simulink model "ksrbl_4k4t_hdtrig"  (Simulink 6.2)
settings: Solver=ode45  StartTime=0.0  StopTime=20000  RelTol=1e-3
libraries: xbsIndex_r3 x1214, casper_library x120, xps_library x20
(part 25 of 26)

== system ksrbl_4k4t_hdtrig/fft_wideband_real/fft_biplex_real_4x0/biplex_core/fft_stage_9/butterfly_direct ==
  a : Inport  Port=1  LatchInput=off
  b : Inport  Port=2  LatchInput=off
  sync : Inport  Port=3  LatchInput=off
  shift : Inport  Port=4  LatchInput=off
  AddSub : xbsIndex_r3/AddSub  mode=Addition  precision=Full  arith_type=Unsigned  n_bits=8  bin_pt=2  quantization=Truncate  overflow=Wrap  latency=add_latency  explicit_period=off  period=1  use_carryin=off  use_carryout=off  en=off  dbl_ovrd=off  show_param=on  use_core=on  pipeline=on  use_rpm=on  gen_core=on
      settings: xl_area=[0, 0, 0, 0, 0, 0, 0]
  AddSub1 : xbsIndex_r3/AddSub  mode=Addition  precision=Full  arith_type=Unsigned  n_bits=8  bin_pt=2  quantization=Truncate  overflow=Wrap  latency=add_latency  explicit_period=off  period=1  use_carryin=off  use_carryout=off  en=off  dbl_ovrd=off  show_param=on  use_core=on  pipeline=on  use_rpm=on  gen_core=on
      settings: xl_area=[0, 0, 0, 0, 0, 0, 0]
  AddSub2 : xbsIndex_r3/AddSub  mode=Subtraction  precision=Full  arith_type=Unsigned  n_bits=8  bin_pt=2  quantization=Truncate  overflow=Wrap  latency=add_latency  explicit_period=off  period=1  use_carryin=off  use_carryout=off  en=off  dbl_ovrd=off  show_param=on  use_core=on  pipeline=on  use_rpm=on  gen_core=on
      settings: xl_area=[0, 0, 0, 0, 0, 0, 0]
  AddSub3 : xbsIndex_r3/AddSub  mode=Subtraction  precision=Full  arith_type=Unsigned  n_bits=8  bin_pt=2  quantization=Truncate  overflow=Wrap  latency=add_latency  explicit_period=off  period=1  use_carryin=off  use_carryout=off  en=off  dbl_ovrd=off  show_param=on  use_core=on  pipeline=on  use_rpm=on  gen_core=on
      settings: xl_area=[0, 0, 0, 0, 0, 0, 0]
  Convert{,1..3} (4 alike) : xbsIndex_r3/Convert  arith_type="Signed  (2's comp)"  n_bits=BitWidth  bin_pt=BitWidth-1  quantization=Truncate  overflow=Wrap  latency=add_latency  explicit_period=off  period=1  dbl_ovrd=off  show_param=off  inserted_by_tool=off  pipeline=off
      settings: xl_area=[0, 0, 0, 0, 0, 0, 0]
  Delay : xbsIndex_r3/Delay  latency=2 * add_latency + 1  reg_retiming=off  explicit_period=off  period=1  en=off  accept_only_valid=off  init_zero=on  dbl_ovrd=off  show_param=off
      settings: xl_area=[0, 0, 0, 0, 0, 0, 0]
  Delay3 : xbsIndex_r3/Delay  latency=1  reg_retiming=off  explicit_period=off  period=1  en=off  accept_only_valid=off  init_zero=on  dbl_ovrd=off  show_param=off
      settings: xl_area=[0, 0, 0, 0, 0, 0, 0]
  Inverter : xbsIndex_r3/Inverter  latency=0  explicit_period=off  period=1  en=off  dbl_ovrd=off  show_param=off
      settings: xl_area=[0, 0, 0, 0, 0, 0, 0]
  Logical : xbsIndex_r3/Logical  logical_function=OR  inputs=4  precision=Full  arith_type=Unsigned  n_bits=8  bin_pt=2  align_bp=on  latency=1  explicit_period=off  period=1  en=off  dbl_ovrd=off  show_param=off
      settings: xl_area=[0, 0, 0, 0, 0, 0, 0]
  Logical{1,4,7,10} (4 alike) : xbsIndex_r3/Logical  logical_function=OR  inputs=2  precision=Full  arith_type=Unsigned  n_bits=8  bin_pt=2  align_bp=off  latency=1  explicit_period=off  period=1  en=off  dbl_ovrd=off  show_param=off
      settings: xl_area=[0, 0, 0, 0, 0, 0, 0]
  Logical{2,5,8,11} (4 alike) : xbsIndex_r3/Logical  logical_function=NOR  inputs=4  precision=Full  arith_type=Unsigned  n_bits=8  bin_pt=2  align_bp=off  latency=1  explicit_period=off  period=1  en=off  dbl_ovrd=off  show_param=off
      settings: xl_area=[0, 0, 0, 0, 0, 0, 0]
  Logical{3,6,9,12} (4 alike) : xbsIndex_r3/Logical  logical_function=AND  inputs=4  precision=Full  arith_type=Unsigned  n_bits=8  bin_pt=2  align_bp=off  latency=1  explicit_period=off  period=1  en=off  dbl_ovrd=off  show_param=off
      settings: xl_area=[0, 0, 0, 0, 0, 0, 0]
  Logical13 : xbsIndex_r3/Logical  logical_function=AND  inputs=2  precision=Full  arith_type=Unsigned  n_bits=8  bin_pt=2  align_bp=off  latency=1  explicit_period=off  period=1  en=off  dbl_ovrd=off  show_param=off
      settings: xl_area=[0, 0, 0, 0, 0, 0, 0]
  Mux{,1..3} (4 alike) : xbsIndex_r3/Mux  inputs=2  precision=Full  arith_type="Signed  (2's comp)"  n_bits=8  bin_pt=2  quantization=Truncate  overflow=Wrap  latency=1  explicit_period=off  period=1  en=off  dbl_ovrd=off  show_param=off  mux_type=off  use_rpm=off  gen_core=off
      settings: xl_area=[0, 0, 0, 0, 0, 0, 0]
  Scale{,1..3} (4 alike) : xbsIndex_r3/Scale  scale_factor=-1  explicit_period=off  period=1  dbl_ovrd=off
  Slice{1,5,9,13} (4 alike) : xbsIndex_r3/Slice  mode=Upper Bit Location + Width  nbits=1  bit1=0  base1=MSB of Input  bit0=0  base0=LSB of Input  boolean_output=on  explicit_period=off  period=1  dbl_ovrd=off
  Slice{2,6,10,14} (4 alike) : xbsIndex_r3/Slice  mode=Upper Bit Location + Width  nbits=1  bit1=-1  base1=MSB of Input  bit0=0  base0=LSB of Input  boolean_output=on  explicit_period=off  period=1  dbl_ovrd=off
  Slice{3,7,11,15} (4 alike) : xbsIndex_r3/Slice  mode=Upper Bit Location + Width  nbits=1  bit1=-2  base1=MSB of Input  bit0=0  base0=LSB of Input  boolean_output=on  explicit_period=off  period=1  dbl_ovrd=off
  Slice{4,8,12,16} (4 alike) : xbsIndex_r3/Slice  mode=Upper Bit Location + Width  nbits=1  bit1=-3  base1=MSB of Input  bit0=0  base0=LSB of Input  boolean_output=on  explicit_period=off  period=1  dbl_ovrd=off
  ri_to_c : casper_library/Misc/ri_to_c
  ri_to_c1 : casper_library/Misc/ri_to_c
  twiddle : Subsystem  BlockChoice=twiddle_general_3mult
      link override twiddle_general_3mult: Coeffs="[1+0i           6.1232e-017-1i               0.70711-0.70711i        -0.70711-0.70711i         0.92388-0.38268i        -0.38268-0.92388i         0.38268-0.92388i        -0.92388-0.38268i         0.98079-0.19509i        -0.19509-0.98079i         0.55557-0.83147i        -0.83147-0.55557i         0.83147-0.55557i        -0.55557-0.83147i         0.19509-0.98079i        -0.98079-0.19509i         0.99518-0.098017i      -0.098017-0.99518i         0.63439-0.77301i        -0.77301-0.63439i         0.88192-0.4714i          -0.4714-0.88192i         0.29028-0.95694i        -0.95694-0.29028i         0.95694-0.29028i        -0.29028-0.95694i          0.4714-0.88192i        -0.88192-0.4714i          0.77301-0.63439i        -0.63439-0.77301i        0.098017-0.99518i        -0.99518-0.098017i         0.9988-0.049068i      -0.049068-0.9988i          0.67156-0.74095i        -0.74095-0.67156i         0.90399-0.42756i        -0.42756-0.90399i         0.33689-0.94154i        -0.94154-0.33689i         0.97003-0.24298i        -0.24298-0.97003i          0.5141-0.85773i        -0.85773-0.5141i          0.80321-0.5957i          -0.5957-0.80321i         0.14673-0.98918i        -0.98918-0.14673i         0.98918-0.14673i        -0.14673-0.98918i          0.5957-0.80321i        -0.80321-0.5957i          0.85773-0.5141i          -0.5141-0.85773i         0.24298-0.97003i        -0.97003-0.24298i         0.94154-0.33689i        -0.33689-0.94154i         0.42756-0.90399i        -0.90399-0.42756i         0.74095-0.67156i        -0.67156-0.74095i        0.049068-0.9988i          -0.9988-0.049068i         0.9997-0.024541i      -0.024541-0.9997i          0.68954-0.72425i        -0.72425-0.68954i         0.91421-0.40524i        -0.40524-0.91421i          0.3599-0.93299i        -0.93299-0.3599i           0.9757-0.2191i          -0.2191-0.9757i            0.535-0.84485i        -0.84485-0.535i           0.81758-0.57581i        -0.57581-0.81758i         0.17096-0.98528i        -0.98528-0.17096i         0.99248-0.12241i        -0.12241-0.99248i         0.61523-0.78835i        -0.78835-0.61523i         0.87009-0.4929i          -0.4929-0.87009i         0.26671-0.96378i        -0.96378-0.26671i         0.94953-0.31368i        -0.31368-0.94953i         0.44961-0.89322i        -0.89322-0.44961i         0.75721-0.65317i        -0.65317-0.75721i        0.073565-0.99729i        -0.99729-0.073565i        0.99729-0.073565i      -0.073565-0.99729i         0.65317-0.75721i        -0.75721-0.65317i         0.89322-0.44961i        -0.44961-0.89322i         0.31368-0.94953i        -0.94953-0.31368i         0.96378-0.26671i        -0.26671-0.96378i          0.4929-0.87009i        -0.87009-0.4929i          0.78835-0.61523i        -0.61523-0.78835i         0.12241-0.99248i        -0.99248-0.12241i         0.98528-0.17096i        -0.17096-0.98528i         0.57581-0.81758i        -0.81758-0.57581i         0.84485-0.535i            -0.535-0.84485i          0.2191-0.9757i          -0.9757-0.2191i          0.93299-0.3599i          -0.3599-0.93299i         0.40524-0.91421i        -0.91421-0.40524i         0.72425-0.68954i        -0.68954-0.72425i        0.024541-0.9997i          -0.9997-0.024541i        0.99992-0.012272i      -0.012272-0.99992i         0.69838-0.71573i        -0.71573-0.69838i         0.91911-0.39399i        -0.39399-0.91911i         0.37132-0.92851i        -0.92851-0.37132i         0.97832-0.20711i        -0.20711-0.97832i         0.54532-0.83822i        -0.83822-0.54532i         0.82459-0.56573i        -0.56573-0.82459i         0.18304-0.98311i        -0.98311-0.18304i         0.99391-0.11022i        -0.11022-0.99391i         0.62486-0.78074i        -0.78074-0.62486i         0.87607-0.48218i        -0.48218-0.87607i         0.27852-0.96043i        -0.96043-0.27852i         0.95331-0.30201i        -0.30201-0.95331i         0.46054-0.88764i        -0.88764-0.46054i         0.76517-0.64383i        -0.64383-0.76517i        0.085797-0.99631i        -0.99631-0.085797i ...(+2393 chars)   ]"  StepPeriod=1  BitWidth=18  add_latency=4  mult_latency=6  bram_latency=4
      link override twiddle_general_3mult/coeff_gen: BlockChoice=br_coeff_gen
      link override twiddle_general_3mult/coeff_gen/br_coeff_gen: Coeffs=[1 2 3 4 5 6 7]  StepPeriod=4  BitWidth=10  bram_latency=6
      link override twiddle_general_3mult/coeff_gen/br_coeff_gen/ROM: distributed_mem=off
      link override twiddle_general_3mult/coeff_gen/br_coeff_gen/ROM1: distributed_mem=off
      link override twiddle_general_3mult/coeff_gen/static_coeff_gen/Constant: equ=P=C
      link override twiddle_general_3mult/coeff_gen/static_coeff_gen/Constant1: equ=P=C
      settings: AttributesFormatString=%<BlockChoice>  TemplateBlock=casper_library/FFTs/Twiddle/twiddle  MemberBlocks=twiddle_coeff_0,twiddle_coeff_1,twiddle_general_3mult,twiddle_general_4mult,twiddle_stage_2
  a+bw : Outport
  a-bw : Outport  Port=2
  of : Outport  Port=3
  sync_out : Outport  Port=4
  wires:
  Inverter/1 -> Logical13/1
  Logical13/1 -> of/1
  Logical/1 -> Logical13/2
  Delay3/1 -> Inverter/1, Mux3/1, Mux2/1, Mux1/1, Mux/1
  Logical7/1 -> Logical/3
  AddSub3/1 -> Scale3/1, Mux3/2
  Logical10/1 -> Logical/4
  Logical11/1 -> Logical10/2
  Logical12/1 -> Logical10/1
  Slice16/1 -> Logical11/3, Logical11/4, Logical12/4
  Slice15/1 -> Logical12/3
  Slice14/1 -> Logical11/2, Logical12/2
  Slice13/1 -> Logical11/1, Logical12/1
  Convert3/1 -> ri_to_c1/2
  Scale3/1 -> Mux3/3
  Mux3/1 -> Slice16/1, Slice15/1, Slice14/1, Slice13/1, Convert3/1
  AddSub2/1 -> Scale2/1, Mux2/2
  Logical8/1 -> Logical7/2
  Logical9/1 -> Logical7/1
  Slice12/1 -> Logical8/4, Logical9/4
  Slice11/1 -> Logical8/3, Logical9/3
  Slice10/1 -> Logical8/2, Logical9/2
  Slice9/1 -> Logical8/1, Logical9/1
  Convert2/1 -> ri_to_c1/1
  Scale2/1 -> Mux2/3
  Mux2/1 -> Slice12/1, Slice11/1, Slice10/1, Slice9/1, Convert2/1
  Logical4/1 -> Logical/2
  Logical5/1 -> Logical4/2
  Logical6/1 -> Logical4/1
  Slice8/1 -> Logical5/3, Logical5/4, Logical6/4
  Slice7/1 -> Logical6/3
  Slice6/1 -> Logical5/2, Logical6/2
  Slice5/1 -> Logical5/1, Logical6/1
  Convert1/1 -> ri_to_c/2
  Scale1/1 -> Mux1/3
  Mux1/1 -> Slice8/1, Slice7/1, Slice6/1, Slice5/1, Convert1/1
  Logical1/1 -> Logical/1
  Logical2/1 -> Logical1/2
  Logical3/1 -> Logical1/1
  Slice4/1 -> Logical2/4, Logical3/4
  Slice3/1 -> Logical2/3, Logical3/3
  Slice2/1 -> Logical2/2, Logical3/2
  Slice1/1 -> Logical2/1, Logical3/1
  Convert/1 -> ri_to_c/1
  Scale/1 -> Mux/3
  Mux/1 -> Slice4/1, Slice3/1, Slice2/1, Slice1/1, Convert/1
  shift/1 -> Delay3/1
  AddSub1/1 -> Scale1/1, Mux1/2
  AddSub/1 -> Scale/1, Mux/2
  Delay/1 -> sync_out/1
  ri_to_c1/1 -> a-bw/1
  ri_to_c/1 -> a+bw/1
  a/1 -> twiddle/1(a)
  b/1 -> twiddle/2(b)
  sync/1 -> twiddle/3(sync)
  twiddle/1(a_re) -> AddSub/1, AddSub2/1
  twiddle/2(a_im) -> AddSub1/1, AddSub3/1
  twiddle/3(bw_re) -> AddSub/2, AddSub2/2
  twiddle/4(bw_im) -> AddSub1/2, AddSub3/2
  twiddle/5(sync_out) -> Delay/1

== system ksrbl_4k4t_hdtrig/fft_wideband_real/fft_biplex_real_4x0/biplex_core/fft_stage_9/delay_b ==
  In1 : Inport  Port=1  LatchInput=off
  delay_slr : casper_library/Delays/delay_slr  DelayLen=2^(FFTSize-FFTStage)
  Out1 : Outport
  wires:
  In1/1 -> delay_slr/1
  delay_slr/1 -> Out1/1

== system ksrbl_4k4t_hdtrig/fft_wideband_real/fft_biplex_real_4x0/biplex_core/fft_stage_9/delay_f ==
  In1 : Inport  Port=1  LatchInput=off
  delay_slr : casper_library/Delays/delay_slr  DelayLen=2^(FFTSize-FFTStage)
  Out1 : Outport
  wires:
  In1/1 -> delay_slr/1
  delay_slr/1 -> Out1/1

== system ksrbl_4k4t_hdtrig/fft_wideband_real/fft_biplex_real_4x0/biplex_core/fft_stage_1/butterfly/c_to_ri ==
  c : Inport  Port=1  LatchInput=off
  Reinterpret : xbsIndex_r3/Reinterpret  force_arith_type=on  arith_type="Signed  (2's comp)"  force_bin_pt=on  bin_pt=BitWidth - 1  force_valid=on
  Reinterpret1 : xbsIndex_r3/Reinterpret  force_arith_type=on  arith_type="Signed  (2's comp)"  force_bin_pt=on  bin_pt=BitWidth - 1  force_valid=on
  Slice : xbsIndex_r3/Slice  mode=Upper Bit Location + Width  nbits=BitWidth  bit1=0  base1=MSB of Input  bit0=0  base0=LSB of Input  boolean_output=off  explicit_period=off  period=1  dbl_ovrd=off
  Slice1 : xbsIndex_r3/Slice  mode=Lower Bit Location + Width  nbits=BitWidth  bit1=0  base1=MSB of Input  bit0=0  base0=LSB of Input  boolean_output=off  explicit_period=off  period=1  dbl_ovrd=off
  re : Outport
  im : Outport  Port=2
  wires:
  Slice/1 -> Reinterpret/1
  Slice1/1 -> Reinterpret1/1
  Reinterpret/1 -> re/1
  Reinterpret1/1 -> im/1
  c/1 -> Slice/1, Slice1/1

== system ksrbl_4k4t_hdtrig/fft_wideband_real/fft_biplex_real_4x0/biplex_core/fft_stage_1/butterfly/c_to_ri1 ==
  c : Inport  Port=1  LatchInput=off
  Reinterpret : xbsIndex_r3/Reinterpret  force_arith_type=on  arith_type="Signed  (2's comp)"  force_bin_pt=on  bin_pt=BitWidth - 1  force_valid=on
  Reinterpret1 : xbsIndex_r3/Reinterpret  force_arith_type=on  arith_type="Signed  (2's comp)"  force_bin_pt=on  bin_pt=BitWidth - 1  force_valid=on
  Slice : xbsIndex_r3/Slice  mode=Upper Bit Location + Width  nbits=BitWidth  bit1=0  base1=MSB of Input  bit0=0  base0=LSB of Input  boolean_output=off  explicit_period=off  period=1  dbl_ovrd=off
  Slice1 : xbsIndex_r3/Slice  mode=Lower Bit Location + Width  nbits=BitWidth  bit1=0  base1=MSB of Input  bit0=0  base0=LSB of Input  boolean_output=off  explicit_period=off  period=1  dbl_ovrd=off
  re : Outport
  im : Outport  Port=2
  wires:
  c/1 -> Slice1/1, Slice/1
  Reinterpret1/1 -> im/1
  Reinterpret/1 -> re/1
  Slice1/1 -> Reinterpret1/1
  Slice/1 -> Reinterpret/1

== system ksrbl_4k4t_hdtrig/fft_wideband_real/fft_biplex_real_4x0/biplex_core/fft_stage_1/butterfly/ri_to_c ==
  re : Inport  Port=1  LatchInput=off
  im : Inport  Port=2  LatchInput=off
  Concat : xbsIndex_r3/Concat  num_inputs=2  explicit_period=off  period=1  dbl_ovrd=off
  Reinterpret : xbsIndex_r3/Reinterpret  force_arith_type=on  arith_type=Unsigned  force_bin_pt=on  bin_pt=0  force_valid=on
  Reinterpret1 : xbsIndex_r3/Reinterpret  force_arith_type=on  arith_type=Unsigned  force_bin_pt=on  bin_pt=0  force_valid=on
  c : Outport
  wires:
  Reinterpret/1 -> Concat/1
  Reinterpret1/1 -> Concat/2
  re/1 -> Reinterpret/1
  Concat/1 -> c/1
  im/1 -> Reinterpret1/1

== system ksrbl_4k4t_hdtrig/fft_wideband_real/fft_biplex_real_4x0/biplex_core/fft_stage_1/butterfly/ri_to_c1 ==
  re : Inport  Port=1  LatchInput=off
  im : Inport  Port=2  LatchInput=off
  Concat : xbsIndex_r3/Concat  num_inputs=2  explicit_period=off  period=1  dbl_ovrd=off
  Reinterpret : xbsIndex_r3/Reinterpret  force_arith_type=on  arith_type=Unsigned  force_bin_pt=on  bin_pt=0  force_valid=on
  Reinterpret1 : xbsIndex_r3/Reinterpret  force_arith_type=on  arith_type=Unsigned  force_bin_pt=on  bin_pt=0  force_valid=on
  c : Outport
  wires:
  Reinterpret/1 -> Concat/1
  Reinterpret1/1 -> Concat/2
  re/1 -> Reinterpret/1
  Concat/1 -> c/1
  im/1 -> Reinterpret1/1

== system ksrbl_4k4t_hdtrig/fft_wideband_real/fft_biplex_real_4x0/biplex_core/fft_stage_10/butterfly_direct/twiddle ==
  a : Inport  Port=1  LatchInput=off
  b : Inport  Port=2  LatchInput=off
  sync : Inport  Port=3  LatchInput=off
  twiddle_general_3mult : casper_library/FFTs/Twiddle/twiddle_general_3mult  Coeffs="[1+0i           6.1232e-017-1i               0.70711-0.70711i        -0.70711-0.70711i         0.92388-0.38268i        -0.38268-0.92388i         0.38268-0.92388i        -0.92388-0.38268i         0.98079-0.19509i        -0.19509-0.98079i         0.55557-0.83147i        -0.83147-0.55557i         0.83147-0.55557i        -0.55557-0.83147i         0.19509-0.98079i        -0.98079-0.19509i         0.99518-0.098017i      -0.098017-0.99518i         0.63439-0.77301i        -0.77301-0.63439i         0.88192-0.4714i          -0.4714-0.88192i         0.29028-0.95694i        -0.95694-0.29028i         0.95694-0.29028i        -0.29028-0.95694i          0.4714-0.88192i        -0.88192-0.4714i          0.77301-0.63439i        -0.63439-0.77301i        0.098017-0.99518i        -0.99518-0.098017i         0.9988-0.049068i      -0.049068-0.9988i          0.67156-0.74095i        -0.74095-0.67156i         0.90399-0.42756i        -0.42756-0.90399i         0.33689-0.94154i        -0.94154-0.33689i         0.97003-0.24298i        -0.24298-0.97003i          0.5141-0.85773i        -0.85773-0.5141i          0.80321-0.5957i          -0.5957-0.80321i         0.14673-0.98918i        -0.98918-0.14673i         0.98918-0.14673i        -0.14673-0.98918i          0.5957-0.80321i        -0.80321-0.5957i          0.85773-0.5141i          -0.5141-0.85773i         0.24298-0.97003i        -0.97003-0.24298i         0.94154-0.33689i        -0.33689-0.94154i         0.42756-0.90399i        -0.90399-0.42756i         0.74095-0.67156i        -0.67156-0.74095i        0.049068-0.9988i          -0.9988-0.049068i         0.9997-0.024541i      -0.024541-0.9997i          0.68954-0.72425i        -0.72425-0.68954i         0.91421-0.40524i        -0.40524-0.91421i          0.3599-0.93299i        -0.93299-0.3599i           0.9757-0.2191i          -0.2191-0.9757i            0.535-0.84485i        -0.84485-0.535i           0.81758-0.57581i        -0.57581-0.81758i         0.17096-0.98528i        -0.98528-0.17096i         0.99248-0.12241i        -0.12241-0.99248i         0.61523-0.78835i        -0.78835-0.61523i         0.87009-0.4929i          -0.4929-0.87009i         0.26671-0.96378i        -0.96378-0.26671i         0.94953-0.31368i        -0.31368-0.94953i         0.44961-0.89322i        -0.89322-0.44961i         0.75721-0.65317i        -0.65317-0.75721i        0.073565-0.99729i        -0.99729-0.073565i        0.99729-0.073565i      -0.073565-0.99729i         0.65317-0.75721i        -0.75721-0.65317i         0.89322-0.44961i        -0.44961-0.89322i         0.31368-0.94953i        -0.94953-0.31368i         0.96378-0.26671i        -0.26671-0.96378i          0.4929-0.87009i        -0.87009-0.4929i          0.78835-0.61523i        -0.61523-0.78835i         0.12241-0.99248i        -0.99248-0.12241i         0.98528-0.17096i        -0.17096-0.98528i         0.57581-0.81758i        -0.81758-0.57581i         0.84485-0.535i            -0.535-0.84485i          0.2191-0.9757i          -0.9757-0.2191i          0.93299-0.3599i          -0.3599-0.93299i         0.40524-0.91421i        -0.91421-0.40524i         0.72425-0.68954i        -0.68954-0.72425i        0.024541-0.9997i          -0.9997-0.024541i        0.99992-0.012272i      -0.012272-0.99992i         0.69838-0.71573i        -0.71573-0.69838i         0.91911-0.39399i        -0.39399-0.91911i         0.37132-0.92851i        -0.92851-0.37132i         0.97832-0.20711i        -0.20711-0.97832i         0.54532-0.83822i        -0.83822-0.54532i         0.82459-0.56573i        -0.56573-0.82459i         0.18304-0.98311i        -0.98311-0.18304i         0.99391-0.11022i        -0.11022-0.99391i         0.62486-0.78074i        -0.78074-0.62486i         0.87607-0.48218i        -0.48218-0.87607i         0.27852-0.96043i        -0.96043-0.27852i         0.95331-0.30201i        -0.30201-0.95331i         0.46054-0.88764i        -0.88764-0.46054i         0.76517-0.64383i        -0.64383-0.76517i        0.085797-0.99631i        -0.99631-0.085797i ...(+8794 chars)  ]"  StepPeriod=0  BitWidth=18  add_latency=4  mult_latency=6  bram_latency=4
  a_re : Outport
  a_im : Outport  Port=2
  bw_re : Outport  Port=3
  bw_im : Outport  Port=4
  sync_out : Outport  Port=5
  wires:
  a/1 -> twiddle_general_3mult/1
  b/1 -> twiddle_general_3mult/2
  sync/1 -> twiddle_general_3mult/3
  twiddle_general_3mult/1 -> a_re/1
  twiddle_general_3mult/2 -> a_im/1
  twiddle_general_3mult/3 -> bw_re/1
  twiddle_general_3mult/4 -> bw_im/1
  twiddle_general_3mult/5 -> sync_out/1

== system ksrbl_4k4t_hdtrig/fft_wideband_real/fft_biplex_real_4x0/biplex_core/fft_stage_2/butterfly_direct/twiddle ==
  a : Inport  Port=1  LatchInput=off
  b : Inport  Port=2  LatchInput=off
  sync : Inport  Port=3  LatchInput=off
  twiddle_stage_2 : casper_library/FFTs/Twiddle/twiddle_stage_2  FFTSize=10  BitWidth=18  add_latency=4  mult_latency=6  bram_latency=4
  a_re : Outport
  a_im : Outport  Port=2
  bw_re : Outport  Port=3
  bw_im : Outport  Port=4
  sync_out : Outport  Port=5
  wires:
  a/1 -> twiddle_stage_2/1
  b/1 -> twiddle_stage_2/2
  sync/1 -> twiddle_stage_2/3
  twiddle_stage_2/1 -> a_re/1
  twiddle_stage_2/2 -> a_im/1
  twiddle_stage_2/3 -> bw_re/1
  twiddle_stage_2/4 -> bw_im/1
  twiddle_stage_2/5 -> sync_out/1

== system ksrbl_4k4t_hdtrig/fft_wideband_real/fft_biplex_real_4x0/biplex_core/fft_stage_3/butterfly_direct/twiddle ==
  a : Inport  Port=1  LatchInput=off
  b : Inport  Port=2  LatchInput=off
  sync : Inport  Port=3  LatchInput=off
  twiddle_general_3mult : casper_library/FFTs/Twiddle/twiddle_general_3mult  Coeffs="[1+0i           6.1232e-017-1i               0.70711-0.70711i        -0.70711-0.70711i    ]"  StepPeriod=7  BitWidth=18  add_latency=4  mult_latency=6  bram_latency=4
  a_re : Outport
  a_im : Outport  Port=2
  bw_re : Outport  Port=3
  bw_im : Outport  Port=4
  sync_out : Outport  Port=5
  wires:
  a/1 -> twiddle_general_3mult/1
  b/1 -> twiddle_general_3mult/2
  sync/1 -> twiddle_general_3mult/3
  twiddle_general_3mult/1 -> a_re/1
  twiddle_general_3mult/2 -> a_im/1
  twiddle_general_3mult/3 -> bw_re/1
  twiddle_general_3mult/4 -> bw_im/1
  twiddle_general_3mult/5 -> sync_out/1

== system ksrbl_4k4t_hdtrig/fft_wideband_real/fft_biplex_real_4x0/biplex_core/fft_stage_4/butterfly_direct/twiddle ==
  a : Inport  Port=1  LatchInput=off
  b : Inport  Port=2  LatchInput=off
  sync : Inport  Port=3  LatchInput=off
  twiddle_general_3mult : casper_library/FFTs/Twiddle/twiddle_general_3mult  Coeffs="[1+0i           6.1232e-017-1i               0.70711-0.70711i        -0.70711-0.70711i         0.92388-0.38268i        -0.38268-0.92388i         0.38268-0.92388i        -0.92388-0.38268i    ]"  StepPeriod=6  BitWidth=18  add_latency=4  mult_latency=6  bram_latency=4
  a_re : Outport
  a_im : Outport  Port=2
  bw_re : Outport  Port=3
  bw_im : Outport  Port=4
  sync_out : Outport  Port=5
  wires:
  a/1 -> twiddle_general_3mult/1
  b/1 -> twiddle_general_3mult/2
  sync/1 -> twiddle_general_3mult/3
  twiddle_general_3mult/1 -> a_re/1
  twiddle_general_3mult/2 -> a_im/1
  twiddle_general_3mult/3 -> bw_re/1
  twiddle_general_3mult/4 -> bw_im/1
  twiddle_general_3mult/5 -> sync_out/1

== system ksrbl_4k4t_hdtrig/fft_wideband_real/fft_biplex_real_4x0/biplex_core/fft_stage_5/butterfly_direct/twiddle ==
  a : Inport  Port=1  LatchInput=off
  b : Inport  Port=2  LatchInput=off
  sync : Inport  Port=3  LatchInput=off
  twiddle_general_3mult : casper_library/FFTs/Twiddle/twiddle_general_3mult  Coeffs="[1+0i           6.1232e-017-1i               0.70711-0.70711i        -0.70711-0.70711i         0.92388-0.38268i        -0.38268-0.92388i         0.38268-0.92388i        -0.92388-0.38268i         0.98079-0.19509i        -0.19509-0.98079i         0.55557-0.83147i        -0.83147-0.55557i         0.83147-0.55557i        -0.55557-0.83147i         0.19509-0.98079i        -0.98079-0.19509i    ]"  StepPeriod=5  BitWidth=18  add_latency=4  mult_latency=6  bram_latency=4
  a_re : Outport
  a_im : Outport  Port=2
  bw_re : Outport  Port=3
  bw_im : Outport  Port=4
  sync_out : Outport  Port=5
  wires:
  a/1 -> twiddle_general_3mult/1
  b/1 -> twiddle_general_3mult/2
  sync/1 -> twiddle_general_3mult/3
  twiddle_general_3mult/1 -> a_re/1
  twiddle_general_3mult/2 -> a_im/1
  twiddle_general_3mult/3 -> bw_re/1
  twiddle_general_3mult/4 -> bw_im/1
  twiddle_general_3mult/5 -> sync_out/1

== system ksrbl_4k4t_hdtrig/fft_wideband_real/fft_biplex_real_4x0/biplex_core/fft_stage_6/butterfly_direct/twiddle ==
  a : Inport  Port=1  LatchInput=off
  b : Inport  Port=2  LatchInput=off
  sync : Inport  Port=3  LatchInput=off
  twiddle_general_3mult : casper_library/FFTs/Twiddle/twiddle_general_3mult  Coeffs="[1+0i           6.1232e-017-1i               0.70711-0.70711i        -0.70711-0.70711i         0.92388-0.38268i        -0.38268-0.92388i         0.38268-0.92388i        -0.92388-0.38268i         0.98079-0.19509i        -0.19509-0.98079i         0.55557-0.83147i        -0.83147-0.55557i         0.83147-0.55557i        -0.55557-0.83147i         0.19509-0.98079i        -0.98079-0.19509i         0.99518-0.098017i      -0.098017-0.99518i         0.63439-0.77301i        -0.77301-0.63439i         0.88192-0.4714i          -0.4714-0.88192i         0.29028-0.95694i        -0.95694-0.29028i         0.95694-0.29028i        -0.29028-0.95694i          0.4714-0.88192i        -0.88192-0.4714i          0.77301-0.63439i        -0.63439-0.77301i        0.098017-0.99518i        -0.99518-0.098017i   ]"  StepPeriod=4  BitWidth=18  add_latency=4  mult_latency=6  bram_latency=4
  a_re : Outport
  a_im : Outport  Port=2
  bw_re : Outport  Port=3
  bw_im : Outport  Port=4
  sync_out : Outport  Port=5
  wires:
  a/1 -> twiddle_general_3mult/1
  b/1 -> twiddle_general_3mult/2
  sync/1 -> twiddle_general_3mult/3
  twiddle_general_3mult/1 -> a_re/1
  twiddle_general_3mult/2 -> a_im/1
  twiddle_general_3mult/3 -> bw_re/1
  twiddle_general_3mult/4 -> bw_im/1
  twiddle_general_3mult/5 -> sync_out/1

== system ksrbl_4k4t_hdtrig/fft_wideband_real/fft_biplex_real_4x0/biplex_core/fft_stage_7/butterfly_direct/twiddle ==
  a : Inport  Port=1  LatchInput=off
  b : Inport  Port=2  LatchInput=off
  sync : Inport  Port=3  LatchInput=off
  twiddle_general_3mult : casper_library/FFTs/Twiddle/twiddle_general_3mult  Coeffs="[1+0i           6.1232e-017-1i               0.70711-0.70711i        -0.70711-0.70711i         0.92388-0.38268i        -0.38268-0.92388i         0.38268-0.92388i        -0.92388-0.38268i         0.98079-0.19509i        -0.19509-0.98079i         0.55557-0.83147i        -0.83147-0.55557i         0.83147-0.55557i        -0.55557-0.83147i         0.19509-0.98079i        -0.98079-0.19509i         0.99518-0.098017i      -0.098017-0.99518i         0.63439-0.77301i        -0.77301-0.63439i         0.88192-0.4714i          -0.4714-0.88192i         0.29028-0.95694i        -0.95694-0.29028i         0.95694-0.29028i        -0.29028-0.95694i          0.4714-0.88192i        -0.88192-0.4714i          0.77301-0.63439i        -0.63439-0.77301i        0.098017-0.99518i        -0.99518-0.098017i         0.9988-0.049068i      -0.049068-0.9988i          0.67156-0.74095i        -0.74095-0.67156i         0.90399-0.42756i        -0.42756-0.90399i         0.33689-0.94154i        -0.94154-0.33689i         0.97003-0.24298i        -0.24298-0.97003i          0.5141-0.85773i        -0.85773-0.5141i          0.80321-0.5957i          -0.5957-0.80321i         0.14673-0.98918i        -0.98918-0.14673i         0.98918-0.14673i        -0.14673-0.98918i          0.5957-0.80321i        -0.80321-0.5957i          0.85773-0.5141i          -0.5141-0.85773i         0.24298-0.97003i        -0.97003-0.24298i         0.94154-0.33689i        -0.33689-0.94154i         0.42756-0.90399i        -0.90399-0.42756i         0.74095-0.67156i        -0.67156-0.74095i        0.049068-0.9988i          -0.9988-0.049068i   ]"  StepPeriod=3  BitWidth=18  add_latency=4  mult_latency=6  bram_latency=4
  a_re : Outport
  a_im : Outport  Port=2
  bw_re : Outport  Port=3
  bw_im : Outport  Port=4
  sync_out : Outport  Port=5
  wires:
  a/1 -> twiddle_general_3mult/1
  b/1 -> twiddle_general_3mult/2
  sync/1 -> twiddle_general_3mult/3
  twiddle_general_3mult/1 -> a_re/1
  twiddle_general_3mult/2 -> a_im/1
  twiddle_general_3mult/3 -> bw_re/1
  twiddle_general_3mult/4 -> bw_im/1
  twiddle_general_3mult/5 -> sync_out/1

== system ksrbl_4k4t_hdtrig/fft_wideband_real/fft_biplex_real_4x0/biplex_core/fft_stage_8/butterfly_direct/twiddle ==
  a : Inport  Port=1  LatchInput=off
  b : Inport  Port=2  LatchInput=off
  sync : Inport  Port=3  LatchInput=off
  twiddle_general_3mult : casper_library/FFTs/Twiddle/twiddle_general_3mult  Coeffs="[1+0i           6.1232e-017-1i               0.70711-0.70711i        -0.70711-0.70711i         0.92388-0.38268i        -0.38268-0.92388i         0.38268-0.92388i        -0.92388-0.38268i         0.98079-0.19509i        -0.19509-0.98079i         0.55557-0.83147i        -0.83147-0.55557i         0.83147-0.55557i        -0.55557-0.83147i         0.19509-0.98079i        -0.98079-0.19509i         0.99518-0.098017i      -0.098017-0.99518i         0.63439-0.77301i        -0.77301-0.63439i         0.88192-0.4714i          -0.4714-0.88192i         0.29028-0.95694i        -0.95694-0.29028i         0.95694-0.29028i        -0.29028-0.95694i          0.4714-0.88192i        -0.88192-0.4714i          0.77301-0.63439i        -0.63439-0.77301i        0.098017-0.99518i        -0.99518-0.098017i         0.9988-0.049068i      -0.049068-0.9988i          0.67156-0.74095i        -0.74095-0.67156i         0.90399-0.42756i        -0.42756-0.90399i         0.33689-0.94154i        -0.94154-0.33689i         0.97003-0.24298i        -0.24298-0.97003i          0.5141-0.85773i        -0.85773-0.5141i          0.80321-0.5957i          -0.5957-0.80321i         0.14673-0.98918i        -0.98918-0.14673i         0.98918-0.14673i        -0.14673-0.98918i          0.5957-0.80321i        -0.80321-0.5957i          0.85773-0.5141i          -0.5141-0.85773i         0.24298-0.97003i        -0.97003-0.24298i         0.94154-0.33689i        -0.33689-0.94154i         0.42756-0.90399i        -0.90399-0.42756i         0.74095-0.67156i        -0.67156-0.74095i        0.049068-0.9988i          -0.9988-0.049068i         0.9997-0.024541i      -0.024541-0.9997i          0.68954-0.72425i        -0.72425-0.68954i         0.91421-0.40524i        -0.40524-0.91421i          0.3599-0.93299i        -0.93299-0.3599i           0.9757-0.2191i          -0.2191-0.9757i            0.535-0.84485i        -0.84485-0.535i           0.81758-0.57581i        -0.57581-0.81758i         0.17096-0.98528i        -0.98528-0.17096i         0.99248-0.12241i        -0.12241-0.99248i         0.61523-0.78835i        -0.78835-0.61523i         0.87009-0.4929i          -0.4929-0.87009i         0.26671-0.96378i        -0.96378-0.26671i         0.94953-0.31368i        -0.31368-0.94953i         0.44961-0.89322i        -0.89322-0.44961i         0.75721-0.65317i        -0.65317-0.75721i        0.073565-0.99729i        -0.99729-0.073565i        0.99729-0.073565i      -0.073565-0.99729i         0.65317-0.75721i        -0.75721-0.65317i         0.89322-0.44961i        -0.44961-0.89322i         0.31368-0.94953i        -0.94953-0.31368i         0.96378-0.26671i        -0.26671-0.96378i          0.4929-0.87009i        -0.87009-0.4929i          0.78835-0.61523i        -0.61523-0.78835i         0.12241-0.99248i        -0.99248-0.12241i         0.98528-0.17096i        -0.17096-0.98528i         0.57581-0.81758i        -0.81758-0.57581i         0.84485-0.535i            -0.535-0.84485i          0.2191-0.9757i          -0.9757-0.2191i          0.93299-0.3599i          -0.3599-0.93299i         0.40524-0.91421i        -0.91421-0.40524i         0.72425-0.68954i        -0.68954-0.72425i        0.024541-0.9997i          -0.9997-0.024541i   ]"  StepPeriod=2  BitWidth=18  add_latency=4  mult_latency=6  bram_latency=4
  a_re : Outport
  a_im : Outport  Port=2
  bw_re : Outport  Port=3
  bw_im : Outport  Port=4
  sync_out : Outport  Port=5
  wires:
  a/1 -> twiddle_general_3mult/1
  b/1 -> twiddle_general_3mult/2
  sync/1 -> twiddle_general_3mult/3
  twiddle_general_3mult/1 -> a_re/1
  twiddle_general_3mult/2 -> a_im/1
  twiddle_general_3mult/3 -> bw_re/1
  twiddle_general_3mult/4 -> bw_im/1
  twiddle_general_3mult/5 -> sync_out/1
